simulink model "B5A4"  (R2015a)
settings: Solver=ode45  StartTime=0.0  StopTime=10.0  RelTol=1e-3
libraries: commchan3 x1, dsparch4 x1, commsink2 x1, commutil2 x1, commfilt2 x1, commrandsrc2 x1, dspsrcs4 x1, dspstat3 x1
settings Model: Creator=Ekko  LastModifiedBy=Ekko

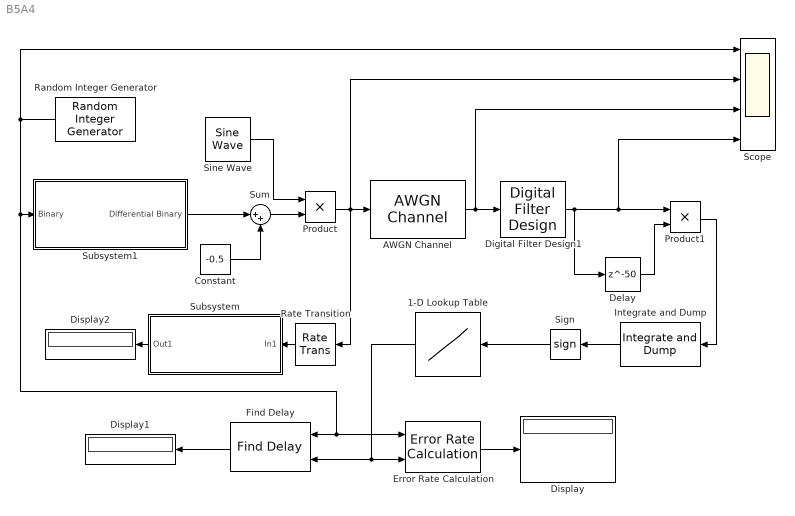
== system B5A4 ==
  1-D Lookup Table : Lookup_n-D  NumberOfTableDimensions=1  BreakpointsForDimension1=[0 1 2 3 4 5]  Table=[-5 -5 -5 -5 0 5]  InternalRulePriority=Speed  RndMeth=Simplest  InputSameDT=on
  AWGN Channel : commchan3/AWGN Channel  InputProcessing=Columns as channels (frame based)  seed=67  noiseMode="Signal to noise ratio  (Eb/No)"  EbNodB=10  EsNodB=10  SNRdB=10  bitsPerSym=1  Ps=1  Tsym=1  variance=1
  Constant : Constant  Value=-0.5  SampleTime=1e-5
  Delay : Delay  DelayLength=50
  Digital Filter Design1 : dsparch4/Digital Filter Design  mwdsp_browser_bugfix_var=off
  Display : Display
  Display1 : Display
  Display2 : Display
  Error Rate Calculation : commsink2/Error Rate Calculation  N=0  st_delay=0  cp_mode=Entire frame  subframe=[]  PMode=Port  WsName=ErrorVec  RsMode2=off  stop=off  numErr=100  maxBits=1e6
  Find Delay : commutil2/Find Delay  corrLength=200  chgSigOP=off  stopUpdate=off  numConstDelay=3
  Integrate and Dump : commfilt2/Integrate and Dump  obssamples=8  offsetsamples=0  nodump=off  roundingMode=Floor  overflowMode=off
  Product : Product
  Product1 : Product
  Random Integer Generator : commrandsrc2/Random Integer Generator  mul=2  seed=37  Ts=1e-5  frameBased=off  sampPerFrame=1  orient=off  outDataType=double
  Rate Transition : RateTransition  Deterministic=off  OutPortSampleTime=1e-5
  Scope : Scope  NumInputPorts=4
      settings: YMin=-5~-5~-5~-5  YMax=5~5~5~5
  Sign : Signum
  Sine Wave : dspsrcs4/Sine Wave  Amplitude=1  Frequency=5000  Phase=0  SampleMode=Discrete  OutComplex=Real  CompMethod=Trigonometric fcn  TableSize=Speed  SampleTime=2e-5  SamplesPerFrame=1  ResetState=Restart at time zero  dataType=double  wordLen=16  udDataType=sfix(16)  fracBitsMode=Best precision  numFracBits=15  OutDataTypeStr=double  LastOutDataTypeStr=double
  Subsystem : Subsystem
  Subsystem1 : Subsystem
  Sum : Sum  Inputs=|++
  wires:
  Subsystem1/1(Differential Binary) -> Sum/1
  Constant/1 -> Sum/2
  Sum/1 -> Product/2
  Sine Wave/1 -> Product/1
  Product/1 -> Scope/2, Rate Transition/1, AWGN Channel/1
  AWGN Channel/1 -> Digital Filter Design1/1, Scope/3
  Digital Filter Design1/1 -> Delay/1, Scope/4, Product1/1
  Delay/1 -> Product1/2
  Product1/1 -> Integrate and Dump/1
  Integrate and Dump/1 -> Sign/1
  Sign/1 -> 1-D Lookup Table/1
  Error Rate Calculation/1 -> Display/1
  Find Delay/1 -> Display1/1
  Subsystem/1(Out1) -> Display2/1
  Rate Transition/1 -> Subsystem/1(In1)
  Random Integer Generator/1 -> Scope/1, Error Rate Calculation/1, Find Delay/1, Subsystem1/1(Binary)
  1-D Lookup Table/1 -> Error Rate Calculation/2, Find Delay/2

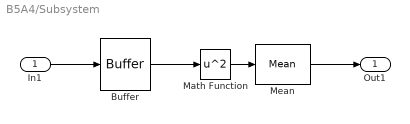
== system B5A4/Subsystem ==
  In1 : Inport
  Buffer : Buffer  TreatMby1Signals=One channel
  Math Function : Math  Operator=square  SaturateOnIntegerOverflow=on
  Mean : dspstat3/Mean  run=off  reset_popup=None  InputProcessing=Columns as channels (frame based)  directionMode=Each column  dimension=1  treatSBRowAsCol=off  roiEnable=off  roiType=Rectangles  roiPortion=Entire ROI  roiOutput=Individual statistics for each ROI  roiFlag=off  outputDataTypeStr=Inherit: Same as accumulator  outputLastDataTypeStr=Inherit: Same as accumulator  outputMin=[]  outputMax=[]  roundingMode=Floor  overflowMode=off
  Out1 : Outport
  wires:
  Buffer/1 -> Math Function/1
  Math Function/1 -> Mean/1
  Mean/1 -> Out1/1
  In1/1 -> Buffer/1

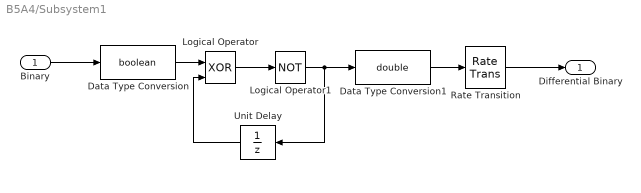
== system B5A4/Subsystem1 ==
  Binary : Inport
  Data Type Conversion : DataTypeConversion  OutDataTypeStr=boolean
  Data Type Conversion1 : DataTypeConversion  OutDataTypeStr=double
  Logical Operator : Logic  Operator=XOR  IconShape=distinctive  AllPortsSameDT=off  OutDataTypeStr=boolean
  Logical Operator1 : Logic  Operator=NOT  IconShape=distinctive  AllPortsSameDT=off  OutDataTypeStr=boolean
  Rate Transition : RateTransition
  Unit Delay : UnitDelay  SampleTime=-1
  Differential Binary : Outport
  wires:
  Rate Transition/1 -> Differential Binary/1
  Data Type Conversion1/1 -> Rate Transition/1
  Data Type Conversion/1 -> Logical Operator/1
  Logical Operator1/1 -> Unit Delay/1, Data Type Conversion1/1
  Binary/1 -> Data Type Conversion/1
  Unit Delay/1 -> Logical Operator/2
  Logical Operator/1 -> Logical Operator1/1
